simulink model "Simulink_asserv"  (R2024a)
settings: Solver=VariableStepAuto  StartTime=0.0  StopTime=10.0  RelTol=1e-3
libraries: simulink x2
settings Model: Creator=alcot161  LastModifiedBy=alcot161

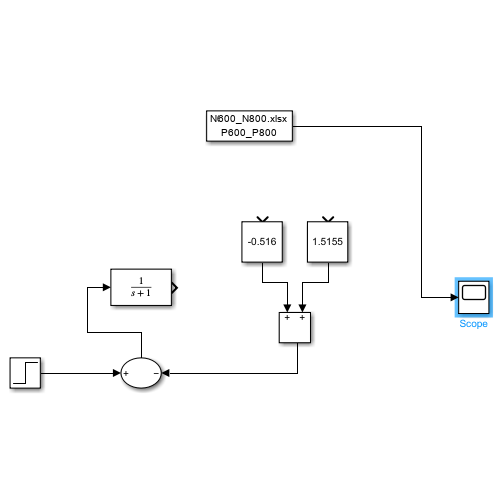
[thumbnail: Simulink's stored preview of the top-level diagram]
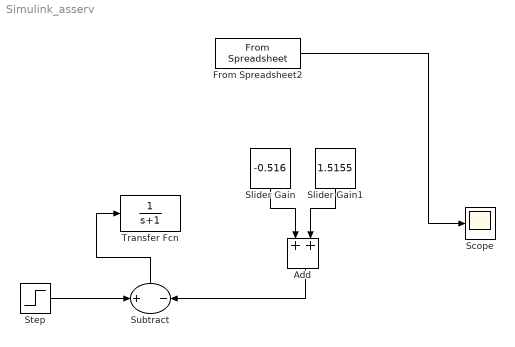
== system Simulink_asserv ==
  Add : Sum
  From Spreadsheet2 : FromSpreadsheet  FileName=N600_N800.xlsx  SheetName=P600_P800  Range=A2:A100  SampleTime=-1
  Scope : Scope
  Slider Gain : simulink/Math Operations/Slider Gain  gain=-0.516  low=-2  high=2
  Slider Gain1 : simulink/Math Operations/Slider Gain  gain=1.5155  low=-2  high=2
  Step : Step  SampleTime=0
  Subtract : Sum  Inputs=+-
  Transfer Fcn : TransferFcn  Denominator=[1 1]
  wires:
  From Spreadsheet2/1 -> Scope/1
  Subtract/1 -> Transfer Fcn/1
  Slider Gain/1 -> Add/1
  Slider Gain1/1 -> Add/2
  Add/1 -> Subtract/2
  Step/1 -> Subtract/1
